simulink model "Cooling_Loop"  (R2022b)
settings: Solver=VariableStepAuto  StartTime=0.0  StopTime=10.0  RelTol=1e-3
settings Model: Creator=spencerdodge  LastModifiedBy=spencerdodge

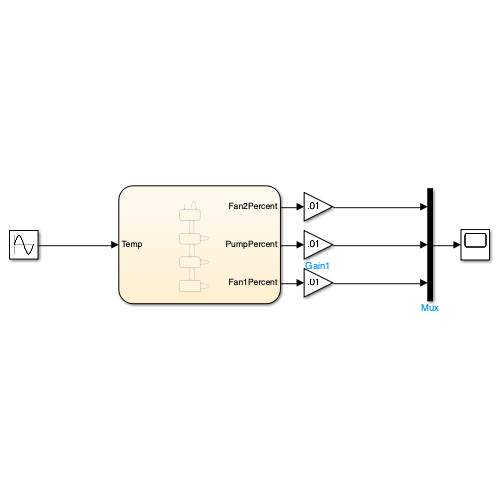
[thumbnail: Simulink's stored preview of the top-level diagram]
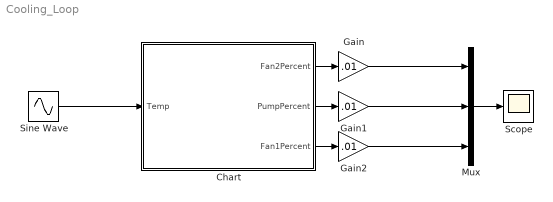
== system Cooling_Loop ==
  Chart : Stateflow chart  TreatAsAtomicUnit=on
  Gain : Gain  Gain=.01
  Gain1 : Gain  Gain=.01
  Gain2 : Gain  Gain=.01
  Mux : Mux  Inputs=3
  Scope : Scope
  Sine Wave : Sin  Amplitude=50  Bias=25  SampleTime=0
  wires:
  Chart/3(Fan1Percent) -> Gain2/1
  Chart/2(PumpPercent) -> Gain1/1
  Chart/1(Fan2Percent) -> Gain/1
  Gain2/1 -> Mux/3
  Gain1/1 -> Mux/2
  Gain/1 -> Mux/1
  Mux/1 -> Scope/1
  Sine Wave/1 -> Chart/1(Temp)

== stateflow chart Cooling_Loop/Chart ==
  state Idle
    PumpPercent = 50;
    Fan1Percent = 0;
    Fan2Percent = 0;
  state Cool_Level_1
    PumpPercent = 50;
    Fan1Percent = 25;
    Fan2Percent = 25;
  state Cool_Level_2
    PumpPercent = 75;
    Fan1Percent = 50;
    Fan2Percent = 50;
  state Cool_Level_Max
    PumpPercent = 100;
    Fan1Percent = 100;
    Fan2Percent = 100;
  Idle -> Idle [order 2] : [Temp < 30]
  (default) -> Idle
  Idle -> Cool_Level_1 [order 1] : [Temp >= 30]
  Cool_Level_1 -> Idle [order 3] : [Temp < 30]
  Cool_Level_1 -> Cool_Level_1 [order 2] : [Temp >= 30]
  Cool_Level_1 -> Cool_Level_2 [order 1] : [Temp >= 40]
  Cool_Level_2 -> Cool_Level_1 [order 3] : [Temp < 40]
  Cool_Level_2 -> Cool_Level_2 [order 2] : [Temp >= 40]
  Cool_Level_2 -> Cool_Level_Max [order 1] : [Temp >= 50]
  Cool_Level_Max -> Cool_Level_2 [order 2] : [Temp < 50]
  Cool_Level_Max -> Cool_Level_Max [order 1] : [Temp >= 50]
  data: Temp input; Fan2Percent output; PumpPercent output; Fan1Percent output
